simulink model "sim_3dof"  (R2025b)
settings: Solver=FixedStepAuto  StartTime=0.0  StopTime=20  FixedStep=0.005  RelTol=1e-3
InitFcn:
  | params_3dof
libraries: simulink_extras x3
settings Model: Creator=schwmaxi  LastModifiedBy=schwmaxi
settings OptimizationCC: UseDivisionForNetSlopeComputation=on  GainParamInheritBuiltInType=on  UseFloatMulNetSlope=on  EnhancedBackFolding=on  BooleansAsBitfields=on  PassReuseOutputArgsAs=Individual arguments  StateBitsets=on  DataBitsets=on  ZeroExternalMemoryAtStartup=off  ZeroInternalMemoryAtStartup=off  NoFixptDivByZeroProtection=on  EfficientFloat2IntCast=on  LifeSpan=1  OptimizeBlockOrder=speed  DifferentSizesBufferReuse=on  EfficientTunableParamExpr=on
settings DebuggingCC: ParameterTunabilityLossMsg=error
settings HardwareCC: ProdBitPerPointer=32.0  ProdBitPerSizeT=32.0  ProdBitPerPtrDiffT=32.0  ProdLargestAtomicFloat=None  ProdWordSize=32.0  ProdLongLongMode=on  ProdHWDeviceType=Custom Processor->Custom Processor
settings SFSimCC: MATLABDynamicMemAlloc=off  SimTargetLang=C++  SimDLTargetLibrary=mkl-dnn
settings RTWCC: SystemTargetFile=ert.tlc  GenCodeOnly=on  TemplateMakefile=ert_default_tmf  TargetLang=C++  Description=Embedded Coder
settings CodeAppCC: ForceParamTrailComments=on  IgnoreCustomStorageClasses=off  OperatorAnnotations=on  SimulinkDataObjDesc=on  SFDataObjDesc=on  CustomSymbolStrGlobalVar=rt$N$M  CustomSymbolStrType=$N$M  CustomSymbolStrFcn=$N$M$F  CustomSymbolStrMacro=$N$M  InsertBlockDesc=on
settings ERTTargetCC: InlinedParameterPlacement=Hierarchical  RootIOFormat=Structure reference  ERTCustomFileTemplate=example_file_process.tlc  ERTFilePackagingFormat=CompactWithDataFile  TargetLangStandard=C++11 (ISO)  GenerateSampleERTMain=on  IncludeMdlTerminateFcn=off  CombineSignalStateStructs=on  SupportAbsoluteTime=off  CodeInterfacePackaging=C++ class  SubcomponentCodeInterfacePackaging=C++ class  SupportComplex=off  SupportNonInlinedSFcns=on

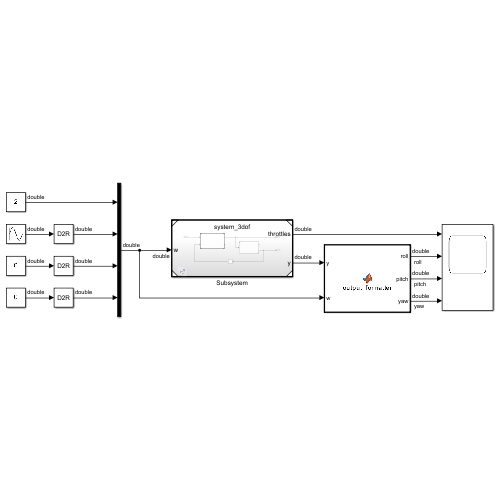
[thumbnail: Simulink's stored preview of the top-level diagram]
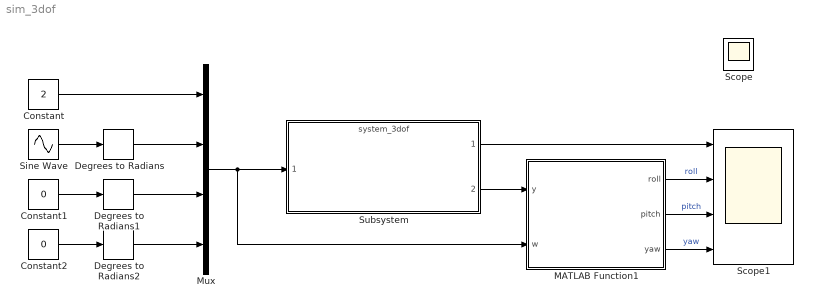
== system sim_3dof ==
  Constant : Constant  Value=2
  Constant1 : Constant  Value=0
  Constant2 : Constant  Value=0
  Degrees to Radians : simulink_extras/Transformations/Degrees to Radians
  Degrees to Radians1 : simulink_extras/Transformations/Degrees to Radians
  Degrees to Radians2 : simulink_extras/Transformations/Degrees to Radians
  MATLAB Function1 : MATLAB Function  TreatAsAtomicUnit=on
  Mux : Mux
  Scope1 : Scope  NumInputPorts=4
      settings: ActiveDisplayString=3  ActiveDisplayYMinimum=-3.1427262187994645E-15  ActiveDisplayYMaximum=3.2624070062908926E-15
  Sine Wave : Sin  Amplitude=3  Frequency=0.2 * 2 * pi  SampleTime=0
  Subsystem : ModelReference  ModelNameDialog=system_3dof  SimulationMode=Normal  ModelReferenceVersion=1.326
  Scope : Scope
      settings: ActiveDisplayYMinimum=-2.1631317412052181E+305  ActiveDisplayYMaximum=4.8211076094254489E+305  DataLoggingVariableName=ScopeData2
  wires:
  Mux/1 -> MATLAB Function1/2(w), Subsystem/1
  Sine Wave/1 -> Degrees to Radians/1
  Constant/1 -> Mux/1
  Constant1/1 -> Degrees to Radians1/1
  Constant2/1 -> Degrees to Radians2/1
  MATLAB Function1/1(roll) -> Scope1/2  "roll"
  MATLAB Function1/2(pitch) -> Scope1/3  "pitch"
  MATLAB Function1/3(yaw) -> Scope1/4  "yaw"
  Degrees to Radians/1 -> Mux/2
  Degrees to Radians1/1 -> Mux/3
  Degrees to Radians2/1 -> Mux/4
  Subsystem/1 -> Scope1/1
  Subsystem/2 -> MATLAB Function1/1(y)

== matlab function sim_3dof/MATLAB Function1 ==
  data: y input; w input; roll output; pitch output; yaw output
function [roll,  pitch, yaw] = output_formatter(y, w)
    y = y * 180 / pi;
    w = w * 180 / pi;

    roll = [w(2), y(1)];
    pitch = [w(3), y(2)];
    yaw = [w(4), y(3)];
end
